simulink model "angular_ctrl"  (R2018a)
settings: Solver=FixedStepAuto  StartTime=0.0  StopTime=inf  MaxStep=0.2  RelTol=1e-3
libraries: arduino_io_lib x5
settings Model: Creator=mhamdi  LastModifiedBy=mhamdi

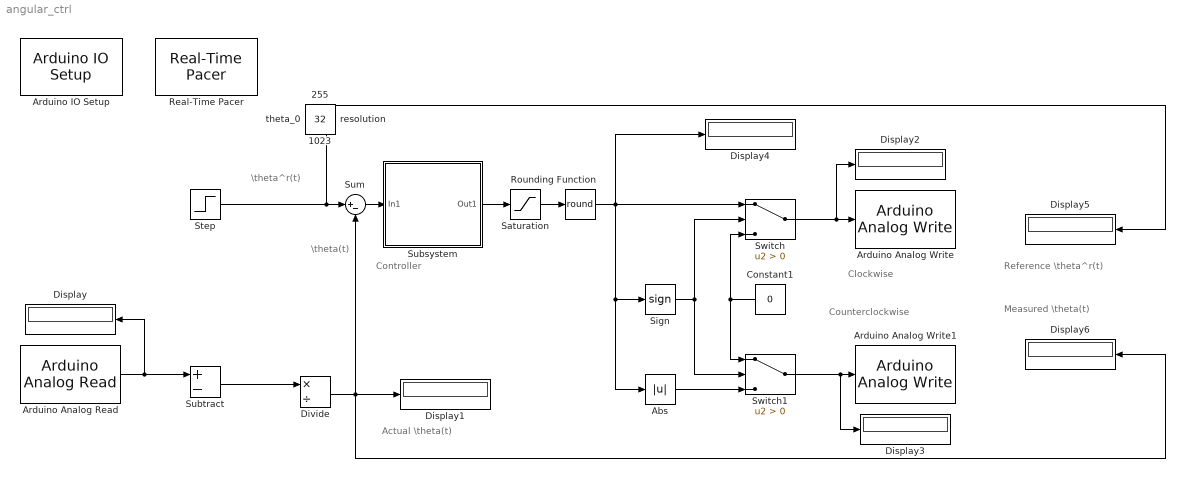
== system angular_ctrl ==
  note: Clockwise
  note: \theta(t)
  note: Counterclockwise
  note: \theta^r(t)
  note: Controller
  note: Actual \theta(t)
  note: Reference \theta^r(t)
  note: Measured \theta(t)
  Abs : Abs
  Arduino Analog Read : arduino_io_lib/Arduino Analog Read  arduinoVar=Temporary arduino variable: Arduino1  arduinoPin=0  T=0.2
  Arduino Analog Write : arduino_io_lib/Arduino Analog Write  arduinoVar=Temporary arduino variable: Arduino1  arduinoPin=5  T=0.2
  Arduino Analog Write1 : arduino_io_lib/Arduino Analog Write  arduinoVar=Temporary arduino variable: Arduino1  arduinoPin=6  T=0.2
  Arduino IO Setup : arduino_io_lib/Arduino IO Setup  Priority=3  arduinoVar=Temporary arduino variable: Arduino1  workspaceVarName=a  comPort=/dev/ttyACM0
  Constant1 : Constant  Value=0
  Display{,1..6} (7 alike) : Display
  Divide : Product  Inputs=*/
  Real-Time Pacer : arduino_io_lib/Real-Time Pacer  simTimePerRealTime=1
  Rounding Function : Rounding  Operator=round
  Saturation : Saturate  UpperLimit=255  LowerLimit=-255
  Sign : Signum
  Step : Step  Time=100  Before=60  After=150  SampleTime=0
  Subsystem : Subsystem  mask{Gr=1.0}
      mask DialogControl DescGroupVar Prompt: Régulateur proportionnel
      mask DialogControl Control2 Prompt: Tournez afin de changer le coefficient du régulateur.
      mask Display: image('/home/mhamdi/MEGA/sci-prod/tbs/elect-cde/lab-elect-cde/imgs/angular/dial_knob.png');
  Subtract : Sum  Inputs=+-
  Sum : Sum  Inputs=|+-
  Switch : Switch  Criteria=u2 > Threshold
  Switch1 : Switch  Criteria=u2 > Threshold
  1023 : Constant  IOType=siggen  Value=1023
  255 : Constant  IOType=siggen  Value=255
  resolution : Constant  IOType=siggen  Value=3.7
  theta_0 : Constant  IOType=siggen  Value=32
  wires:
  Arduino Analog Read/1 -> Subtract/1, Display/1
  Subtract/1 -> Divide/1
  Divide/1 -> Sum/2, Display6/1, Display1/1
  Sign/1 -> Switch1/2, Switch/2
  Switch1/1 -> Arduino Analog Write1/1, Display3/1
  Switch/1 -> Arduino Analog Write/1, Display2/1
  Abs/1 -> Switch1/3
  Constant1/1 -> Switch1/1, Switch/3
  Saturation/1 -> Rounding Function/1
  Rounding Function/1 -> Sign/1, Abs/1, Switch/1, Display4/1
  Sum/1 -> Subsystem/1(In1)
  Subsystem/1(Out1) -> Saturation/1
  Step/1 -> Sum/1, Display5/1

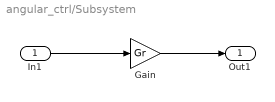
== system angular_ctrl/Subsystem ==
  In1 : Inport
  Gain : Gain  Gain=Gr
  Out1 : Outport
  wires:
  Gain/1 -> Out1/1
  In1/1 -> Gain/1
